simulink model "PID_controlinput_disturbance_delay"  (R2022a)
settings: Solver=VariableStepAuto  StartTime=0.0  StopTime=0.1  RelTol=1e-3
libraries: cstblocks x4
settings Model: Creator=Linxi Ren  LastModifiedBy=Linxi Ren

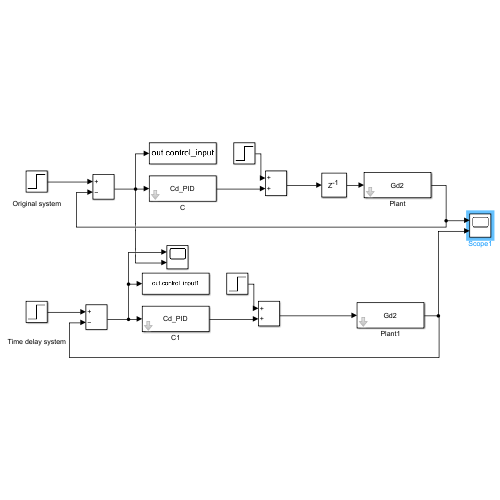
[thumbnail: Simulink's stored preview of the top-level diagram]
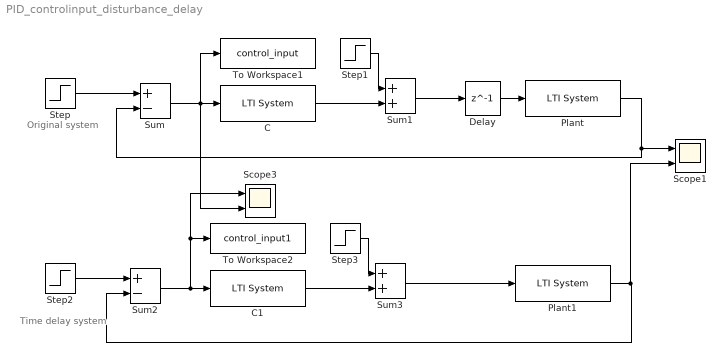
== system PID_controlinput_disturbance_delay ==
  note: Time delay system
  note: Original system
  C : cstblocks/LTI System  sys=Cd_PID  IC=[]
  C1 : cstblocks/LTI System  sys=Cd_PID  IC=[]
  Delay : Delay  DelayLength=1  InitialCondition=0
  Plant : cstblocks/LTI System  sys=Gd2  IC=[]
  Plant1 : cstblocks/LTI System  sys=Gd2  IC=[]
  Scope1 : Scope  NumInputPorts=2
  Scope3 : Scope  NumInputPorts=2
  Step : Step  Time=0  After=0  SampleTime=0
  Step1 : Step  Time=0  SampleTime=0.0005
  Step2 : Step  Time=0  After=0  SampleTime=0
  Step3 : Step  Time=0  SampleTime=0.0005
  Sum : Sum  Inputs=+-  InputSameDT=on  SaturateOnIntegerOverflow=on  OutDataTypeStr=Inherit: Same as first input
  Sum1 : Sum  InputSameDT=on  SaturateOnIntegerOverflow=on  OutDataTypeStr=Inherit: Same as first input
  Sum2 : Sum  Inputs=+-  InputSameDT=on  SaturateOnIntegerOverflow=on  OutDataTypeStr=Inherit: Same as first input
  Sum3 : Sum  InputSameDT=on  SaturateOnIntegerOverflow=on  OutDataTypeStr=Inherit: Same as first input
  To Workspace1 : ToWorkspace  VariableName=control_input  SaveFormat=Timeseries  SampleTime=-1
  To Workspace2 : ToWorkspace  VariableName=control_input1  SaveFormat=Timeseries  SampleTime=-1
  wires:
  Step/1 -> Sum/1
  C/1 -> Sum1/2
  Plant/1 -> Scope1/1, Sum/2
  Step1/1 -> Sum1/1
  Sum/1 -> Scope3/2, To Workspace1/1, C/1
  Delay/1 -> Plant/1
  Sum1/1 -> Delay/1
  Sum2/1 -> Scope3/1, To Workspace2/1, C1/1
  Plant1/1 -> Scope1/2, Sum2/2
  Step2/1 -> Sum2/1
  Step3/1 -> Sum3/1
  C1/1 -> Sum3/2
  Sum3/1 -> Plant1/1
